simulink model "HilClimbers_Integrated_V8_2018b"  (R2018b)
settings: Solver=VariableStepAuto  StartTime=0.0  StopTime=20  RelTol=1e-3
undefined symbols (not defined in the file): air_conditioner_on_value, car_efficiency, op_type, sigbuilder_block, temperature_conversion, zero_check
libraries: BCM x10, simulink x2
settings Model: Creator=achu  LastModifiedBy=achu
settings DataIOCC: ReturnWorkspaceOutputs=on
settings DebuggingCC: AlgebraicLoopMsg=none  ParameterPrecisionLossMsg=none  SFMachineParentedDataDiag=error

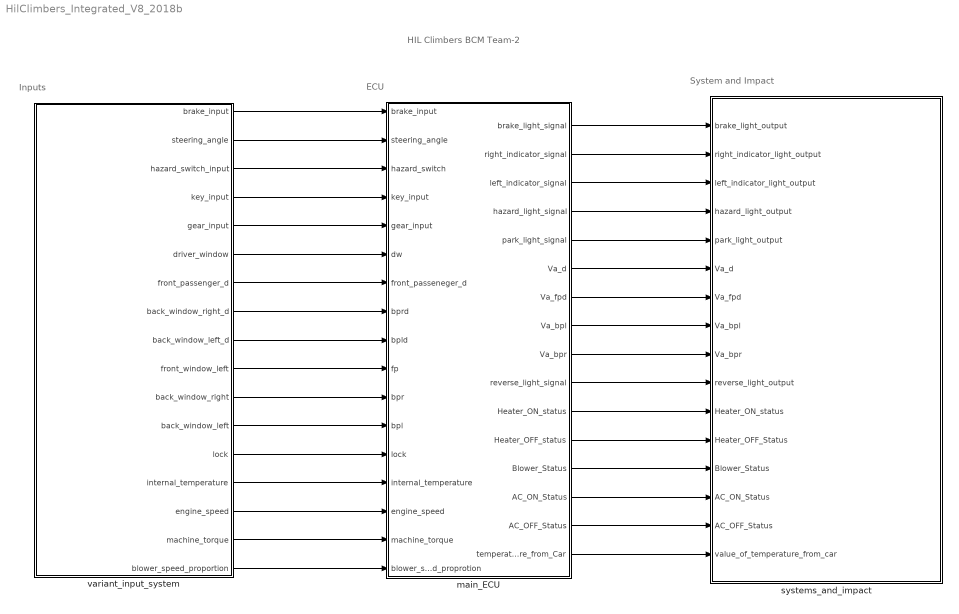
== system HilClimbers_Integrated_V8_2018b ==
  note: HIL Climbers BCM Team-2
  note: Inputs
  note: ECU
  note: System and Impact
  main_ECU : Subsystem
  systems_and_impact : Subsystem
  variant_input_system : Subsystem  Variant=on
  wires:
  main_ECU/3(left_indicator_signal) -> systems_and_impact/3(left_indicator_light_output)
  variant_input_system/13(lock) -> main_ECU/13(lock)
  variant_input_system/5(gear_input) -> main_ECU/5(gear_input)
  main_ECU/11(Heater_ON_status) -> systems_and_impact/11(Heater_ON_status)
  variant_input_system/9(back_window_left_d) -> main_ECU/9(bpld)
  variant_input_system/2(steering_angle) -> main_ECU/2(steering_angle)
  main_ECU/2(right_indicator_signal) -> systems_and_impact/2(right_indicator_light_output)
  variant_input_system/17(blower_speed_proportion) -> main_ECU/17(blower_speed_proprotion)
  main_ECU/16(temperature_from_Car) -> systems_and_impact/16(value_of_temperature_from_car)
  variant_input_system/12(back_window_left) -> main_ECU/12(bpl)
  main_ECU/15(AC_OFF_Status) -> systems_and_impact/15(AC_OFF_Status)
  variant_input_system/6(driver_window) -> main_ECU/6(dw)
  variant_input_system/7(front_passenger_d) -> main_ECU/7(front_passeneger_d)
  variant_input_system/16(machine_torque) -> main_ECU/16(machine_torque)
  main_ECU/4(hazard_light_signal) -> systems_and_impact/4(hazard_light_output)
  main_ECU/8(Va_bpl) -> systems_and_impact/8(Va_bpl)
  variant_input_system/15(engine_speed) -> main_ECU/15(engine_speed)
  main_ECU/10(reverse_light_signal) -> systems_and_impact/10(reverse_light_output)
  main_ECU/13(Blower_Status) -> systems_and_impact/13(Blower_Status)
  variant_input_system/3(hazard_switch_input) -> main_ECU/3(hazard_switch)
  main_ECU/14(AC_ON_Status) -> systems_and_impact/14(AC_ON_Status)
  variant_input_system/8(back_window_right_d) -> main_ECU/8(bprd)
  variant_input_system/14(internal_temperature) -> main_ECU/14(internal_temperature)
  variant_input_system/4(key_input) -> main_ECU/4(key_input)
  variant_input_system/1(brake_input) -> main_ECU/1(brake_input)
  main_ECU/6(Va_d) -> systems_and_impact/6(Va_d)
  variant_input_system/11(back_window_right) -> main_ECU/11(bpr)
  variant_input_system/10(front_window_left) -> main_ECU/10(fp)
  main_ECU/7(Va_fpd) -> systems_and_impact/7(Va_fpd)
  main_ECU/12(Heater_OFF_status) -> systems_and_impact/12(Heater_OFF_Status)
  main_ECU/1(brake_light_signal) -> systems_and_impact/1(brake_light_output)
  main_ECU/9(Va_bpr) -> systems_and_impact/9(Va_bpr)
  main_ECU/5(park_light_signal) -> systems_and_impact/5(park_light_output)

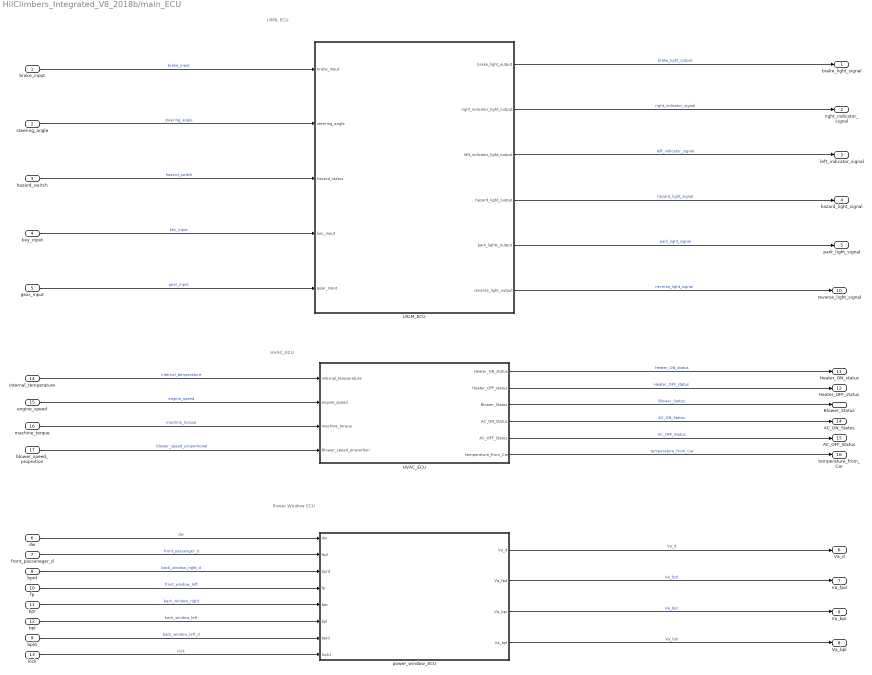
== system HilClimbers_Integrated_V8_2018b/main_ECU ==
  note: Power Window ECU
  note: HVAC_ECU
  note: LRML ECU
  brake_input : Inport
  steering_angle : Inport  Port=2
  hazard_switch : Inport  Port=3
  key_input : Inport  Port=4
  gear_input : Inport  Port=5
  dw : Inport  Port=6
  front_passeneger_d : Inport  Port=7
  bprd : Inport  Port=8
  bpld : Inport  Port=9
  fp : Inport  Port=10
  bpr : Inport  Port=11
  bpl : Inport  Port=12
  lock : Inport  Port=13
  internal_temperature : Inport  Port=14
  engine_speed : Inport  Port=15
  machine_torque : Inport  Port=16
  blower_speed_proprotion : Inport  Port=17
  HVAC_ECU : Subsystem
  LRLM_ECU : Subsystem
  power_window_ECU : Subsystem
  brake_light_signal : Outport
  right_indicator_signal : Outport  Port=2
  left_indicator_signal : Outport  Port=3
  hazard_light_signal : Outport  Port=4
  park_light_signal : Outport  Port=5
  Va_d : Outport  Port=6
  Va_fpd : Outport  Port=7
  Va_bpl : Outport  Port=8
  Va_bpr : Outport  Port=9
  reverse_light_signal : Outport  Port=10
  Heater_ON_status : Outport  Port=11
  Heater_OFF_status : Outport  Port=12
  Blower_Status : Outport  Port=13
  AC_ON_Status : Outport  Port=14
  AC_OFF_Status : Outport  Port=15
  temperature_from_Car : Outport  Port=16
  wires:
  HVAC_ECU/1(Heater_ON_status) -> Heater_ON_status/1  "Heater_ON_status"
  hazard_switch/1 -> LRLM_ECU/3(hazard_status)  "hazard_switch"
  LRLM_ECU/1(brake_light_output) -> brake_light_signal/1  "brake_light_output"
  HVAC_ECU/5(AC_OFF_Status) -> AC_OFF_Status/1  "AC_OFF_Status"
  steering_angle/1 -> LRLM_ECU/2(steering_angle)  "steering_angle"
  LRLM_ECU/2(right_indicator_light_output) -> right_indicator_signal/1  "right_indicator_signal"
  LRLM_ECU/5(park_lights_output) -> park_light_signal/1  "park_light_signal"
  brake_input/1 -> LRLM_ECU/1(brake_input)  "brake_input"
  engine_speed/1 -> HVAC_ECU/2(engine_speed)  "engine_speed"
  LRLM_ECU/3(left_indicator_light_output) -> left_indicator_signal/1  "left_indicator_signal"
  LRLM_ECU/4(hazard_light_output) -> hazard_light_signal/1  "hazard_light_signal"
  internal_temperature/1 -> HVAC_ECU/1(internal_temperature)  "internal_temperature"
  LRLM_ECU/6(reverse_light_output) -> reverse_light_signal/1  "reverse_light_signal"
  gear_input/1 -> LRLM_ECU/5(gear_input)  "gear_input"
  HVAC_ECU/2(Heater_OFF_status) -> Heater_OFF_status/1  "Heater_OFF_status"
  key_input/1 -> LRLM_ECU/4(key_input)  "key_input"
  blower_speed_proprotion/1 -> HVAC_ECU/4(Blower_speed_proportion)  "blower_speed_proportional"
  HVAC_ECU/6(temperature_from_Car) -> temperature_from_Car/1  "temperature_from_Car"
  HVAC_ECU/4(AC_ON_Status) -> AC_ON_Status/1  "AC_ON_Status"
  machine_torque/1 -> HVAC_ECU/3(machine_torque)  "machine_torque"
  HVAC_ECU/3(Blower_Status) -> Blower_Status/1  "Blower_Status"
  power_window_ECU/1(Va_d) -> Va_d/1  "Va_d"
  bpl/1 -> power_window_ECU/6(bpl)  "back_window_left"
  power_window_ECU/3(Va_bpr) -> Va_bpr/1  "Va_bpr"
  bpld/1 -> power_window_ECU/7(bpld)  "back_window_left_d"
  bprd/1 -> power_window_ECU/3(bprd)  "back_window_right_d"
  fp/1 -> power_window_ECU/4(fp)  "front_window_left"
  power_window_ECU/2(Va_fpd) -> Va_fpd/1  "Va_fpd"
  bpr/1 -> power_window_ECU/5(bpr)  "back_window_right"
  dw/1 -> power_window_ECU/1(dw)  "dw"
  power_window_ECU/4(Va_bpl) -> Va_bpl/1  "Va_bpl"
  lock/1 -> power_window_ECU/8(lock1)  "lock"
  front_passeneger_d/1 -> power_window_ECU/2(fpd)  "front_passenger_d"

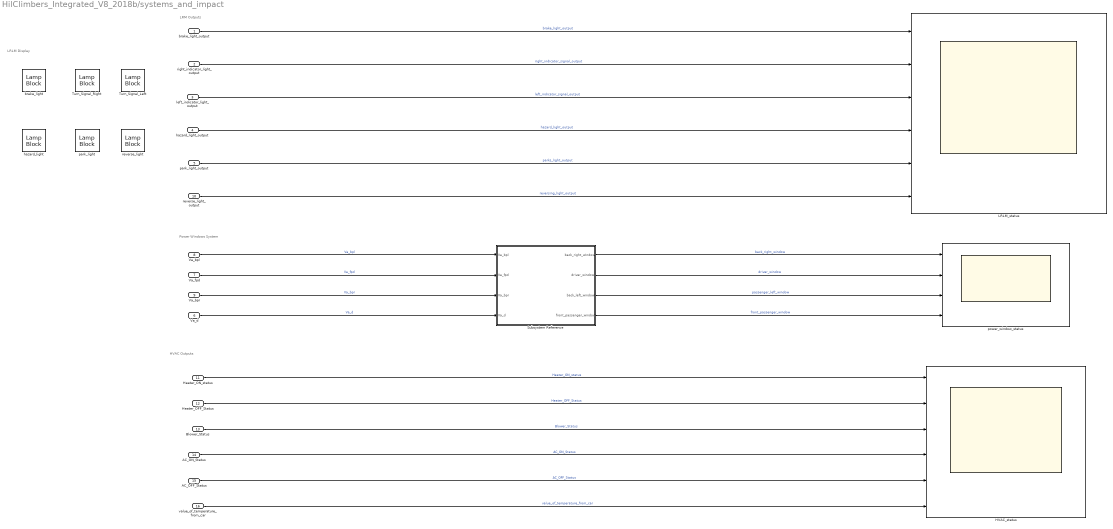
== system HilClimbers_Integrated_V8_2018b/systems_and_impact ==
  note: HVAC Outputs
  note: Power Windows System
  note: LRM Outputs
  note: LRLM Display
  brake_light_output : Inport
  right_indicator_light_output : Inport  Port=2
  left_indicator_light_output : Inport  Port=3
  hazard_light_output : Inport  Port=4
  park_light_output : Inport  Port=5
  Va_d : Inport  Port=6
  Va_fpd : Inport  Port=7
  Va_bpl : Inport  Port=8
  Va_bpr : Inport  Port=9
  reverse_light_output : Inport  Port=10
  Heater_ON_status : Inport  Port=11
  Heater_OFF_Status : Inport  Port=12
  Blower_Status : Inport  Port=13
  AC_ON_Status : Inport  Port=14
  AC_OFF_Status : Inport  Port=15
  value_of_temperature_from_car : Inport  Port=16
  HVAC_status : Scope  NumInputPorts=6
  LRLM_status : Scope  NumInputPorts=6
  Subsystem Reference : Subsystem
  Turn_Signal_Left : LampBlock  LabelPosition=Hide  Icon=TurnSignalLeft  WebBlockId=61
  Turn_Signal_Right : LampBlock  LabelPosition=Hide  Icon=TurnSignalRight  WebBlockId=62
  brake_light : LampBlock  LabelPosition=Hide  Icon=LightingSwitch  WebBlockId=63
  hazard_light : LampBlock  LabelPosition=Hide  Icon=Hazards  WebBlockId=64
  park_light : LampBlock  LabelPosition=Hide  Icon=ParkingAssistance  WebBlockId=65
  power_window_status : Scope  NumInputPorts=4
  reverse_light : LampBlock  LabelPosition=Hide  Icon=RearFogLight  WebBlockId=67
  wires:
  hazard_light_output/1 -> LRLM_status/4  "hazard_light_output"
  reverse_light_output/1 -> LRLM_status/6  "reversing_light_output"
  park_light_output/1 -> LRLM_status/5  "parks_light_output"
  left_indicator_light_output/1 -> LRLM_status/3  "left_indicator_signal_output"
  right_indicator_light_output/1 -> LRLM_status/2  "right_indicator_signal_output"
  brake_light_output/1 -> LRLM_status/1  "brake_light_output"
  Subsystem Reference/4(front_passenger_window) -> power_window_status/4  "front_passenger_window"
  Subsystem Reference/3(back_left_window) -> power_window_status/3  "passenger_left_window"
  Subsystem Reference/1(back_right_window) -> power_window_status/1  "back_right_window"
  Subsystem Reference/2(driver_window) -> power_window_status/2  "driver_window"
  Blower_Status/1 -> HVAC_status/3  "Blower_Status"
  AC_OFF_Status/1 -> HVAC_status/5  "AC_OFF_Status"
  AC_ON_Status/1 -> HVAC_status/4  "AC_ON_Status"
  Heater_OFF_Status/1 -> HVAC_status/2  "Heater_OFF_Status"
  Heater_ON_status/1 -> HVAC_status/1  "Heater_ON_status"
  value_of_temperature_from_car/1 -> HVAC_status/6  "value_of_temperature_from_car"
  Va_bpl/1 -> Subsystem Reference/1(Va_bpl)  "Va_bpl"
  Va_fpd/1 -> Subsystem Reference/2(Va_fpd)  "Va_fpd"
  Va_d/1 -> Subsystem Reference/4(Va_d)  "Va_d"
  Va_bpr/1 -> Subsystem Reference/3(Va_bpr)  "Va_bpr"

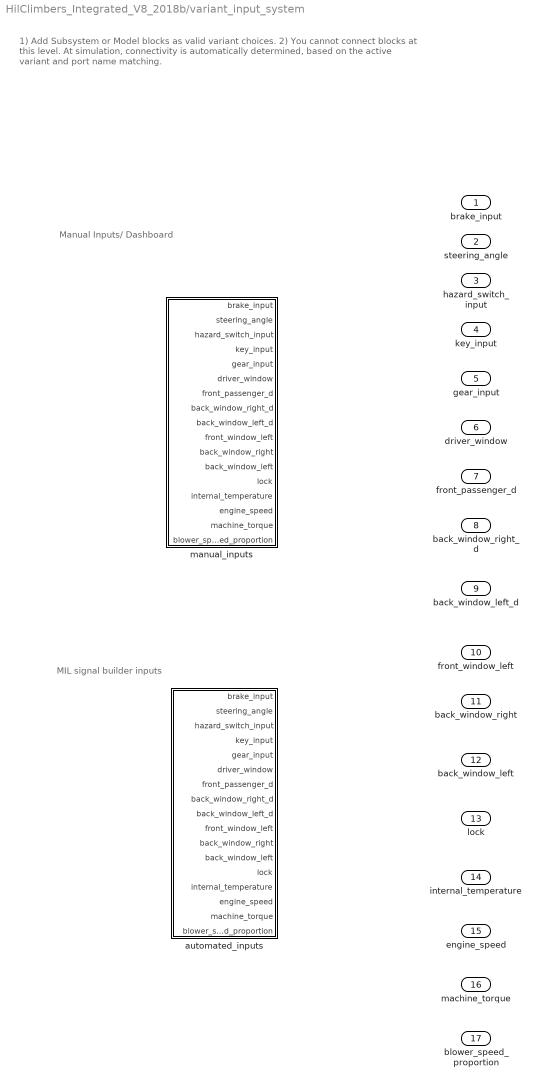
== system HilClimbers_Integrated_V8_2018b/variant_input_system ==
  note: MIL signal builder inputs
  note: Manual Inputs/ Dashboard
  note: 1) Add Subsystem or Model blocks as valid variant choices.
      | 2) You cannot connect blocks at this level. At simulation, connectivity is automatically
      | determined, based on the active variant and port name matching.
  automated_inputs : Subsystem  VariantControl=automated_input
  manual_inputs : Subsystem  VariantControl=manual_input
  brake_input : Outport
  steering_angle : Outport  Port=2
  hazard_switch_input : Outport  Port=3
  key_input : Outport  Port=4
  gear_input : Outport  Port=5
  driver_window : Outport  Port=6
  front_passenger_d : Outport  Port=7
  back_window_right_d : Outport  Port=8
  back_window_left_d : Outport  Port=9
  front_window_left : Outport  Port=10
  back_window_right : Outport  Port=11
  back_window_left : Outport  Port=12
  lock : Outport  Port=13
  internal_temperature : Outport  Port=14
  engine_speed : Outport  Port=15
  machine_torque : Outport  Port=16
  blower_speed_proportion : Outport  Port=17

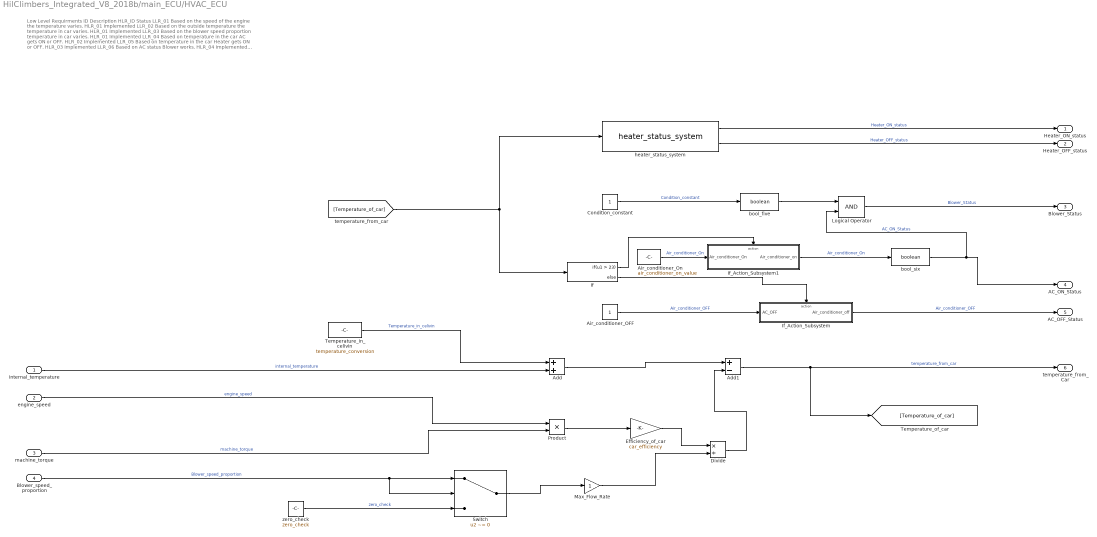
== system HilClimbers_Integrated_V8_2018b/main_ECU/HVAC_ECU ==
  note: Low Level Requirments
      | ID
      | Description
      | HLR_ID
      | Status
      |
      | LLR_01
      | Based on the speed of the engine the temperature varies.
      | HLR_01
      | Implemented
      |
      | LLR_02
      | Based on the outside temperature the temperature in car varies.
      | HLR_01
      | Implemented
      |
      | LLR_03
      | Based on the blower speed proportion temperature in car varies.
      | HLR_01
      | Implemented
      |
      | LLR_04
      | Based on temperature in the car AC gets ON or OFF.
      | HLR_02
      | Implemented
      |
      | LLR_05
      | Based on temperature in the car Heater gets ON or OFF.
      | HLR_03
      | Implemented
      |
      | LLR_06
      | Based on AC status Blower works.
      | HLR_04
      | Implemented
      |
      | LOGIC:
      | STEP 1. Taking values of engine temperature and comp Torque and multipled and given to efficiency(gain).
      | STEP 2. Blower speed proportion and given toMaximum flow rate(gain).
      | STEP 3. Both values were given to divide block.
      | STEP 4. Internal Temperature is in degrees and after it converted into kelvin.
      | STEP 5. Subtract of both values, then the temperature will display on the Display block.
      | 1.Based on temperature the AC is getting on.
      | a.If the value(temperature) is greater than 23 then AC should be on.
      | b.Else the AC should be off.
      | 2. Based on AC status Blower Works.
      | 3. Based on temperature the Blower is getting on.
      | a.If the value(temperature) is less than 18 then Heater should be on.
      | b.Else the Heater should be off.
  internal_temperature : Inport
  engine_speed : Inport  Port=2
  machine_torque : Inport  Port=3
  Blower_speed_proportion : Inport  Port=4
  Add : Sum
  Add1 : Sum  Inputs=+-
  Air_conditioner_OFF : Constant
  Air_conditioner_On : Constant  Value=air_conditioner_on_value
  Condition_constant : Constant
  Divide : Product  Inputs=*/
  Efficiency_of_car : Gain  Gain=car_efficiency
  If : If  IfExpression=u1 > 23
  If_Action_Subsystem : Subsystem  TreatAsAtomicUnit=on
  If_Action_Subsystem1 : Subsystem  TreatAsAtomicUnit=on
  Logical Operator : Logic  AllPortsSameDT=off  OutDataTypeStr=boolean
  Max_Flow_Rate : Gain
  Product : Product
  Switch : Switch  Criteria=u2 ~= 0
  Temperature_in_celivin : Constant  Value=temperature_conversion
  bool_five : DataTypeConversion  OutDataTypeStr=boolean
  bool_six : DataTypeConversion  OutDataTypeStr=boolean
  heater_status_system : BCM/heater_status_system  SystemSampleTime=-1  Latency=0  AutoFrameSizeCalculation=off
      settings: SourceProductName=BCM Library
  zero_check : Constant  Value=zero_check
  Heater_ON_status : Outport
  Heater_OFF_status : Outport  Port=2
  Blower_Status : Outport  Port=3
  AC_ON_Status : Outport  Port=4
  AC_OFF_Status : Outport  Port=5
  temperature_from_Car : Outport  Port=6
  wires:
  Add1/1 -> temperature_from_Car/1, [Temperature_of_car]  "temperature_from_car"
  If_Action_Subsystem/1(Air_conditioner_off) -> AC_OFF_Status/1  "Air_conditioner_OFF"
  Divide/1 -> Add1/2
  [Temperature_of_car] -> heater_status_system/1, If/1
  Condition_constant/1 -> bool_five/1  "Condition_constant"
  Efficiency_of_car/1 -> Divide/1
  If/1 -> If_Action_Subsystem1/Action
  Air_conditioner_OFF/1 -> If_Action_Subsystem/1(AC_OFF)  "Air_conditioner_OFF"
  Max_Flow_Rate/1 -> Divide/2
  Add/1 -> Add1/1
  Temperature_in_celivin/1 -> Add/1  "Temperature_in_celivin"
  engine_speed/1 -> Product/1  "engine_speed"
  machine_torque/1 -> Product/2  "machine_torque"
  internal_temperature/1 -> Add/2  "internal_temperature"
  If/2 -> If_Action_Subsystem/Action
  Product/1 -> Efficiency_of_car/1
  Logical Operator/1 -> Blower_Status/1  "Blower_Status"
  Air_conditioner_On/1 -> If_Action_Subsystem1/1(Air_conditioner_On)  "Air_conditioner_On"
  heater_status_system/1 -> Heater_ON_status/1  "Heater_ON_status"
  heater_status_system/2 -> Heater_OFF_status/1  "Heater_OFF_status"
  Switch/1 -> Max_Flow_Rate/1
  Blower_speed_proportion/1 -> Switch/1, Switch/2  "Blower_speed_proportion"
  bool_five/1 -> Logical Operator/1
  If_Action_Subsystem1/1(Air_conditioner_on) -> bool_six/1  "Air_conditioner_On"
  bool_six/1 -> Logical Operator/2, AC_ON_Status/1  "AC_ON_Status"
  zero_check/1 -> Switch/3  "zero_check"

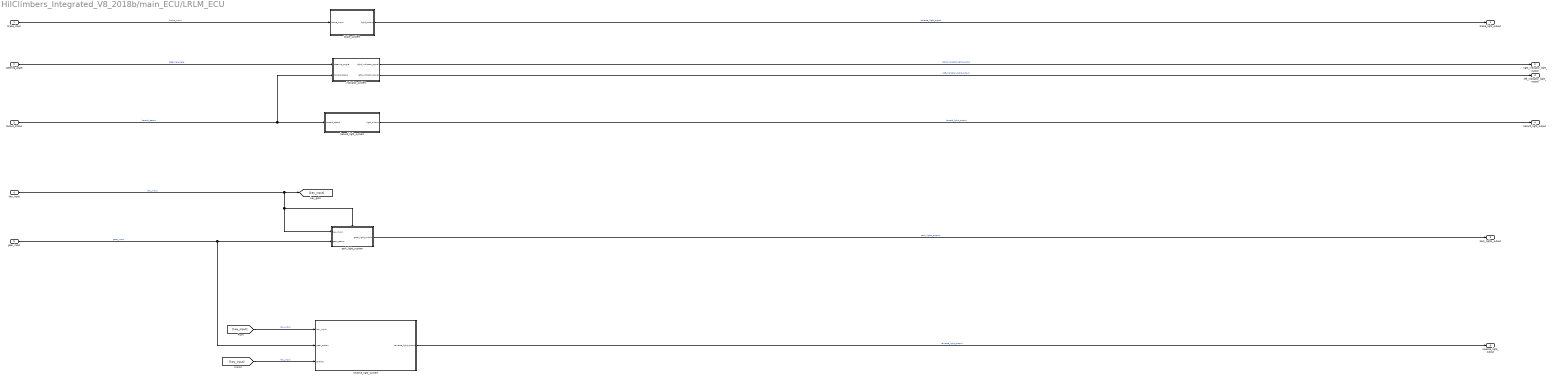
== system HilClimbers_Integrated_V8_2018b/main_ECU/LRLM_ECU ==
  brake_input : Inport
  steering_angle : Inport  Port=2
  hazard_status : Inport  Port=3
  key_input : Inport  Port=4
  gear_input : Inport  Port=5
  brake_system : Subsystem  TreatAsAtomicUnit=on
      mask Display: disp("Brake System");
  hazard_light_system : Subsystem
  indicator_system : Subsystem  TreatAsAtomicUnit=on
  park_light_system : Subsystem
  reverse_light_system : Subsystem  Variant=on
  brake_light_output : Outport
  right_indicator_light_output : Outport  Port=2
  left_indicator_light_output : Outport  Port=3
  hazard_light_output : Outport  Port=4
  park_lights_output : Outport  Port=5
  reverse_light_output : Outport  Port=6
  wires:
  hazard_light_system/1(light_output) -> hazard_light_output/1  "hazard_light_output"
  brake_input/1 -> brake_system/1(brake_input)  "brake_input"
  park_light_system/1(gear_light_output) -> park_lights_output/1  "park_lights_output"
  hazard_status/1 -> indicator_system/2(hazard_status), hazard_light_system/1(hazard_status)  "hazard_status"
  indicator_system/2(left_indicator_signal) -> left_indicator_light_output/1  "left_indicator_light_output"
  indicator_system/1(right_indicator_signal) -> right_indicator_light_output/1  "right_indicator_light_output"
  steering_angle/1 -> indicator_system/1(steering_angle)  "steering_angle"
  brake_system/1(light_output) -> brake_light_output/1  "reverse_light_signal"
  gear_input/1 -> reverse_light_system/2(gear_option), park_light_system/2(gear_status)  "gear_input"
  key_input/1 -> park_light_system/Enable, park_light_system/1(key_input), [key_input]  "key_input"
  [key_input] -> reverse_light_system/1(key_input)  "key_input"
  [key_input] -> reverse_light_system/3(Enable)  "key_input"
  reverse_light_system/1(reverse_light_output) -> reverse_light_output/1  "reverse_light_output"

== system HilClimbers_Integrated_V8_2018b/main_ECU/power_window_ECU ==
  dw : Inport
  fpd : Inport  Port=2
  bprd : Inport  Port=3
  fp : Inport  Port=4
  bpr : Inport  Port=5
  bpl : Inport  Port=6
  bpld : Inport  Port=7
  lock1 : Inport  Port=8
  Checking_priority : Subsystem  TreatAsAtomicUnit=on
  MATLAB Function4 : MATLAB Function  TreatAsAtomicUnit=on
  Va_d : Outport
  Va_fpd : Outport  Port=2
  Va_bpr : Outport  Port=3
  Va_bpl : Outport  Port=4
  wires:
  MATLAB Function4/2(Va_fpd) -> Va_fpd/1  "Va_fpd"
  MATLAB Function4/3(Va_bpr) -> Va_bpr/1  "Va_bpr"
  lock1/1 -> Checking_priority/5(lock)  "lock"
  fpd/1 -> Checking_priority/1(fpd)  "fpd"
  bpld/1 -> Checking_priority/4(bpld)  "bpld"
  MATLAB Function4/1(Va_d) -> Va_d/1  "Va_d"
  Checking_priority/1(front_passenger) -> MATLAB Function4/2(front_passenger)  "front_passenger"
  dw/1 -> MATLAB Function4/1(dw)  "dw"
  bpl/1 -> Checking_priority/3(bpl)  "bpl"
  Checking_priority/2(back_passenger_right) -> MATLAB Function4/3(back_passenger_right)  "back_passenger_right"
  fp/1 -> Checking_priority/7(fp)  "fp"
  bpr/1 -> Checking_priority/6(bpr)  "bpr"
  bprd/1 -> Checking_priority/2(bprd)  "bprd"
  Checking_priority/3(back_passenger_left) -> MATLAB Function4/4(back_passenger_left)  "back_passenger_left"
  MATLAB Function4/4(Va_bpl) -> Va_bpl/1  "Va_bpl"

== system HilClimbers_Integrated_V8_2018b/systems_and_impact/Subsystem Reference ==
  Va_bpl : Inport
  Va_fpd : Inport  Port=2
  Va_bpr : Inport  Port=3
  Va_d : Inport  Port=4
  MATLAB Function : MATLAB Function  TreatAsAtomicUnit=on
  power_window_dc_motor{,1..3} (4 alike) : BCM/power_window_dc_motor  SystemSampleTime=-1  Latency=0  AutoFrameSizeCalculation=off
      settings: SourceProductName=BCM Library
  back_right_window : Outport
  driver_window : Outport  Port=2
  back_left_window : Outport  Port=3
  front_passenger_window : Outport  Port=4
  wires:
  Va_fpd/1 -> power_window_dc_motor3/2, power_window_dc_motor3/1  "Va_fpd"
  Va_d/1 -> power_window_dc_motor1/2, power_window_dc_motor1/1  "Va_d"
  power_window_dc_motor3/1 -> MATLAB Function/4(fp)
  power_window_dc_motor1/1 -> MATLAB Function/2(d)  "d"
  MATLAB Function/1(pr_o) -> back_right_window/1  "back_right_window"
  power_window_dc_motor/1 -> MATLAB Function/1(pr)
  Va_bpr/1 -> power_window_dc_motor/2, power_window_dc_motor/1  "Va_bpr"
  MATLAB Function/2(d_o) -> driver_window/1  "driver_window"
  MATLAB Function/3(pl_o) -> back_left_window/1  "back_left_window"
  MATLAB Function/4(fp_o) -> front_passenger_window/1  "front_passenger_window"
  Va_bpl/1 -> power_window_dc_motor2/2, power_window_dc_motor2/1  "Va_bpl"
  power_window_dc_motor2/1 -> MATLAB Function/3(pl)  "d"

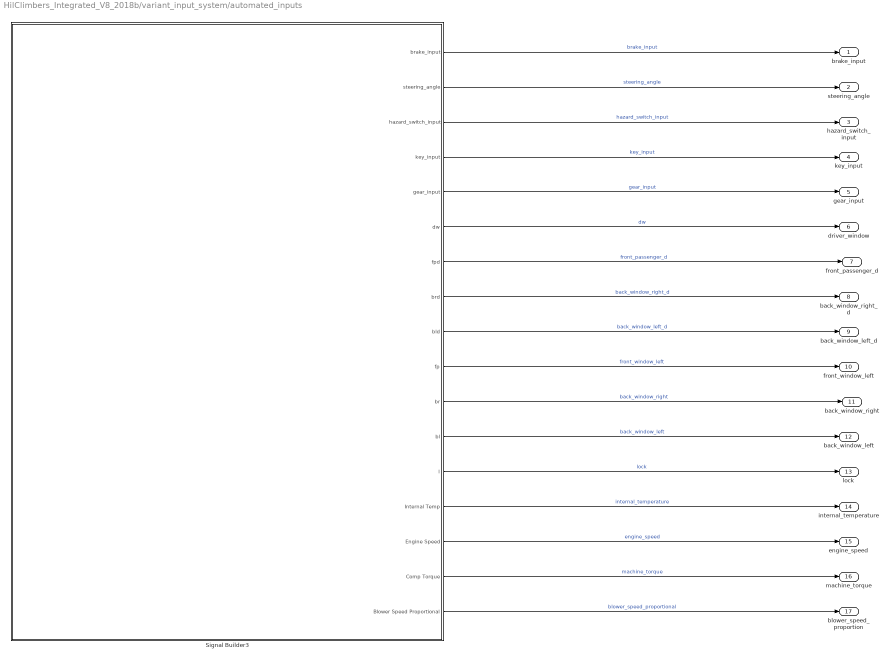
== system HilClimbers_Integrated_V8_2018b/variant_input_system/automated_inputs ==
  Signal Builder3 : Subsystem  Tag=STV Subsys  LoadFcn=sigbuilder_block('load');  StartFcn=sigbuilder_block('start');  StopFcn=sigbuilder_block('stop');  ClipboardFcn=sigbuilder_block('clipboard');  mask(Sigbuilder block){tuvar=[0:10]}
      mask help: Simulink:masks:SigbuilderBlock_MD
      mask init:
      | if ~strcmp(get_param(bdroot(gcbh),'SimulationStatus'),'stopped') tuvar = sigbuilder_block('maskInit'); end
      settings: CopyFcn=sigbuilder_block('copy');  DeleteFcn=sigbuilder_block('delete');  ModelCloseFcn=sigbuilder_block('modelClose');  PreSaveFcn=sigbuilder_block('preSave');  PauseFcn=sigbuilder_block('pause');  ContinueFcn=sigbuilder_block('continue');  NameChangeFcn=sigbuilder_block('namechange');  OpenFcn=sigbuilder_block('open',[437.6 199.2 550.4 400 ]);  CloseFcn=sigbuilder_block('close');
      mask Display: plot(0, 0, 100, 100,[2, 2, 32, 32, 2], [68, 8, 8, 68, 68],[32, 2], [38, 38], [32, 19, 2],[53, 60, 44], [32, 17, 17, 2],[16, 16, 31, 31]);txt = getActiveGroup(gcbh);text(2, 100, txt,'verticalAlignment', 'top');
  brake_input : Outport
  steering_angle : Outport  Port=2
  hazard_switch_input : Outport  Port=3
  key_input : Outport  Port=4
  gear_input : Outport  Port=5
  driver_window : Outport  Port=6
  front_passenger_d : Outport  Port=7
  back_window_right_d : Outport  Port=8
  back_window_left_d : Outport  Port=9
  front_window_left : Outport  Port=10
  back_window_right : Outport  Port=11
  back_window_left : Outport  Port=12
  lock : Outport  Port=13
  internal_temperature : Outport  Port=14
  engine_speed : Outport  Port=15
  machine_torque : Outport  Port=16
  blower_speed_proportion : Outport  Port=17
  wires:
  Signal Builder3/11(br) -> back_window_right/1  "back_window_right"
  Signal Builder3/2(steering_angle) -> steering_angle/1  "steering_angle"
  Signal Builder3/13(l) -> lock/1  "lock"
  Signal Builder3/16(Comp Torque) -> machine_torque/1  "machine_torque"
  Signal Builder3/10(fp) -> front_window_left/1  "front_window_left"
  Signal Builder3/5(gear_input) -> gear_input/1  "gear_input"
  Signal Builder3/12(bl) -> back_window_left/1  "back_window_left"
  Signal Builder3/17(Blower Speed Proportional) -> blower_speed_proportion/1  "blower_speed_proportional"
  Signal Builder3/8(brd) -> back_window_right_d/1  "back_window_right_d"
  Signal Builder3/14(Internal Temp) -> internal_temperature/1  "internal_temperature"
  Signal Builder3/3(hazard_switch_input) -> hazard_switch_input/1  "hazard_switch_input"
  Signal Builder3/6(dw) -> driver_window/1  "dw"
  Signal Builder3/1(brake_input) -> brake_input/1  "brake_input"
  Signal Builder3/7(fpd) -> front_passenger_d/1  "front_passenger_d"
  Signal Builder3/9(bld) -> back_window_left_d/1  "back_window_left_d"
  Signal Builder3/15(Engine Speed) -> engine_speed/1  "engine_speed"
  Signal Builder3/4(key_input) -> key_input/1  "key_input"

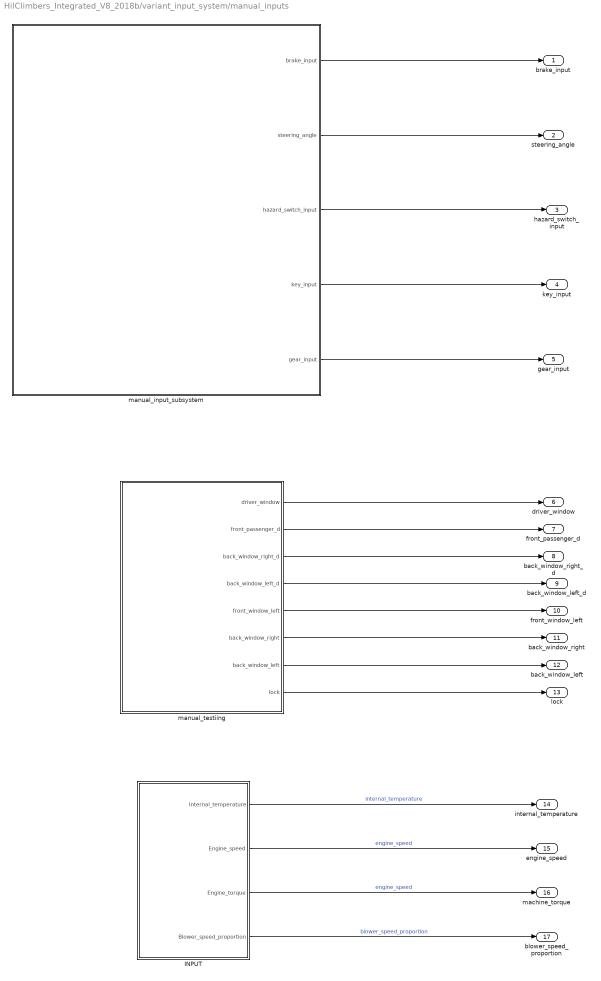
== system HilClimbers_Integrated_V8_2018b/variant_input_system/manual_inputs ==
  INPUT : Subsystem
  manual_input_subsystem : Subsystem  VariantControl=manual_test
  manual_testiing : Subsystem  VariantControl=Choice
  brake_input : Outport
  steering_angle : Outport  Port=2
  hazard_switch_input : Outport  Port=3
  key_input : Outport  Port=4
  gear_input : Outport  Port=5
  driver_window : Outport  Port=6
  front_passenger_d : Outport  Port=7
  back_window_right_d : Outport  Port=8
  back_window_left_d : Outport  Port=9
  front_window_left : Outport  Port=10
  back_window_right : Outport  Port=11
  back_window_left : Outport  Port=12
  lock : Outport  Port=13
  internal_temperature : Outport  Port=14
  engine_speed : Outport  Port=15
  machine_torque : Outport  Port=16
  blower_speed_proportion : Outport  Port=17
  wires:
  manual_input_subsystem/3(hazard_switch_input) -> hazard_switch_input/1
  manual_input_subsystem/2(steering_angle) -> steering_angle/1
  manual_input_subsystem/4(key_input) -> key_input/1
  manual_testiing/1(driver_window) -> driver_window/1
  manual_input_subsystem/1(brake_input) -> brake_input/1
  manual_testiing/6(back_window_right) -> back_window_right/1
  manual_testiing/5(front_window_left) -> front_window_left/1
  manual_input_subsystem/5(gear_input) -> gear_input/1
  manual_testiing/3(back_window_right_d) -> back_window_right_d/1
  INPUT/1(Internal_temperature) -> internal_temperature/1  "internal_temperature"
  manual_testiing/8(lock) -> lock/1
  INPUT/3(Engine_torque) -> machine_torque/1  "engine_speed"
  manual_testiing/4(back_window_left_d) -> back_window_left_d/1
  INPUT/2(Engine_speed) -> engine_speed/1  "engine_speed"
  manual_testiing/2(front_passenger_d) -> front_passenger_d/1
  INPUT/4(Blower_speed_proportion) -> blower_speed_proportion/1  "blower_speed_proportion"
  manual_testiing/7(back_window_left) -> back_window_left/1

== system HilClimbers_Integrated_V8_2018b/main_ECU/HVAC_ECU/If_Action_Subsystem ==
  AC_OFF : Inport
  Action_Port : ActionPort
  Air_conditioner_off : Outport
  wires:
  AC_OFF/1 -> Air_conditioner_off/1  "AC_OFF"

== system HilClimbers_Integrated_V8_2018b/main_ECU/HVAC_ECU/If_Action_Subsystem1 ==
  Air_conditioner_On : Inport
  Action_Port : ActionPort
  Air_conditioner_on : Outport
  wires:
  Air_conditioner_On/1 -> Air_conditioner_on/1  "Air_conditioner_On"

== system HilClimbers_Integrated_V8_2018b/main_ECU/LRLM_ECU/brake_system ==
  brake_input : Inport
  brake/hazard_light_output_decider : BCM/brake//hazard_light_output_decider
      settings: SourceProductName=BCM Library
  light_output : Outport
  wires:
  brake_input/1 -> brake/hazard_light_output_decider/1  "brake_input"
  brake/hazard_light_output_decider/1 -> light_output/1

== system HilClimbers_Integrated_V8_2018b/main_ECU/LRLM_ECU/hazard_light_system ==
  hazard_status : Inport
  brake/hazard_light_output_decider : BCM/brake//hazard_light_output_decider
      settings: SourceProductName=BCM Library
  light_output : Outport
  wires:
  brake/hazard_light_output_decider/1 -> light_output/1  "light_output"
  hazard_status/1 -> brake/hazard_light_output_decider/1  "hazard_switch_input"

== system HilClimbers_Integrated_V8_2018b/main_ECU/LRLM_ECU/indicator_system ==
  steering_angle : Inport
  hazard_status : Inport  Port=2
  left_indicator_system : Subsystem
  right_indicator_system : Subsystem
  right_indicator_signal : Outport
  left_indicator_signal : Outport  Port=2
  wires:
  left_indicator_system/1(left_indicator_signal) -> left_indicator_signal/1  "left_indicator_signal"
  right_indicator_system/1(right_indicator_signal) -> right_indicator_signal/1  "right_indicator_signal"
  hazard_status/1 -> right_indicator_system/2(hazard_status), left_indicator_system/2(hazard_status)  "hazard_status"
  steering_angle/1 -> right_indicator_system/1(steering_angle), [steering_angle]  "steering_angle"
  [steering_angle] -> left_indicator_system/1(steering_angle)  "steering_angle"

== system HilClimbers_Integrated_V8_2018b/main_ECU/LRLM_ECU/park_light_system ==
  key_input : Inport
  gear_status : Inport  Port=2
  Enable : EnablePort  StatesWhenEnabling=reset
  bool_fourty : DataTypeConversion  OutDataTypeStr=boolean
  bool_fourtyone : DataTypeConversion  OutDataTypeStr=boolean
  park_gear_lights_output_decider : BCM/reverse//park_gear_lights_output_decider  gear_option=Park
      settings: SourceProductName=BCM Library
  gear_light_output : Outport
  wires:
  bool_fourty/1 -> park_gear_lights_output_decider/1
  bool_fourtyone/1 -> park_gear_lights_output_decider/2
  key_input/1 -> bool_fourty/1  "key_input"
  gear_status/1 -> bool_fourtyone/1  "gear_status"
  park_gear_lights_output_decider/1 -> gear_light_output/1  "gear_light_output"

== system HilClimbers_Integrated_V8_2018b/main_ECU/LRLM_ECU/reverse_light_system ==
  note: 1) Add Subsystem or Model blocks as valid variant choices.
      | 2) You cannot connect blocks at this level. At simulation, connectivity is automatically
      | determined, based on the active variant and port name matching.
  key_input : Inport
  gear_option : Inport  Port=2
  Enable : Inport  Port=3
  reverse_light_mil : Subsystem  TreatAsAtomicUnit=on  VariantControl=reverse_light_sys_mil  mask{out_type=Reverse lights will blink}
      mask prompts: out_type "Enter the mode of reverse lights"
      mask init:
      | assignin('base','op_type',out_type);
      mask TypeOptions out_type: Reverse lights will blink | Reverse lights will not blink
  reverse_light_sil : Subsystem  VariantControl=reverse_light_sys_sil  mask{sfcnParam1=op_type}
      mask prompts: sfcnParam1 "op_type:"
      mask help: Simulink:masks:GenSFuncDesc_MD
      mask Help: eval('feval(''rtwprivate'',''rtwhelpview'',''rtw_sfcn_block'')');
  reverse_light_output : Outport

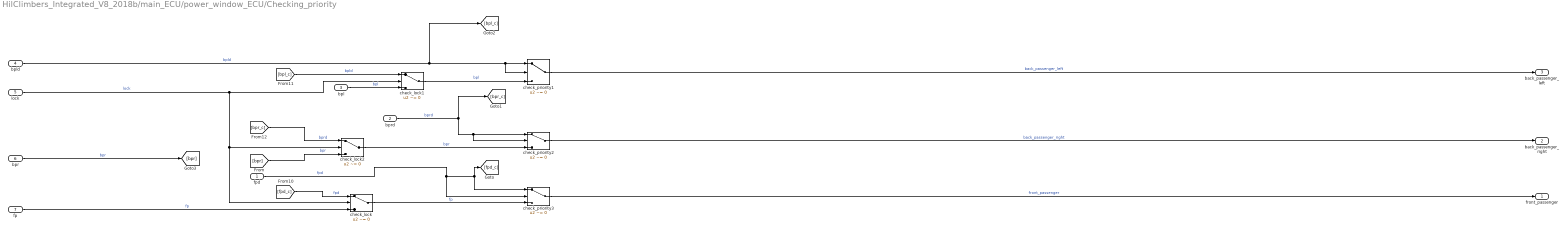
== system HilClimbers_Integrated_V8_2018b/main_ECU/power_window_ECU/Checking_priority ==
  fpd : Inport
  bprd : Inport  Port=2
  bpl : Inport  Port=3
  bpld : Inport  Port=4
  lock : Inport  Port=5
  bpr : Inport  Port=6
  fp : Inport  Port=7
  check_lock : Switch  Criteria=u2 ~= 0
  check_lock1 : Switch  Criteria=u2 ~= 0
  check_lock2 : Switch  Criteria=u2 ~= 0
  check_priority1 : Switch  Criteria=u2 ~= 0
  check_priority2 : Switch  Criteria=u2 ~= 0
  check_priority3 : Switch  Criteria=u2 ~= 0
  front_passenger : Outport
  back_passenger_right : Outport  Port=2
  back_passenger_left : Outport  Port=3
  wires:
  check_lock2/1 -> check_priority2/3  "bpr"
  bprd/1 -> check_priority2/2, check_priority2/1, [bpr_c]  "bprd"
  bpld/1 -> [bpl_c], check_priority1/1, check_priority1/2  "bpld"
  check_priority1/1 -> back_passenger_left/1  "back_passenger_left"
  check_priority2/1 -> back_passenger_right/1  "back_passenger_right"
  check_priority3/1 -> front_passenger/1  "front_passenger"
  lock/1 -> check_lock/2, check_lock2/2, check_lock1/2  "lock"
  bpl/1 -> check_lock1/3  "bpl"
  check_lock1/1 -> check_priority1/3  "bpl"
  [bpl_c] -> check_lock1/1  "bpld"
  [fpd_c] -> check_lock/1  "fpd"
  [bpr] -> check_lock2/3  "bpr"
  [bpr_c] -> check_lock2/1  "bprd"
  bpr/1 -> [bpr]  "bpr"
  fp/1 -> check_lock/3  "fp"
  fpd/1 -> check_priority3/2, [fpd_c], check_priority3/1  "fpd"
  check_lock/1 -> check_priority3/3  "fp"

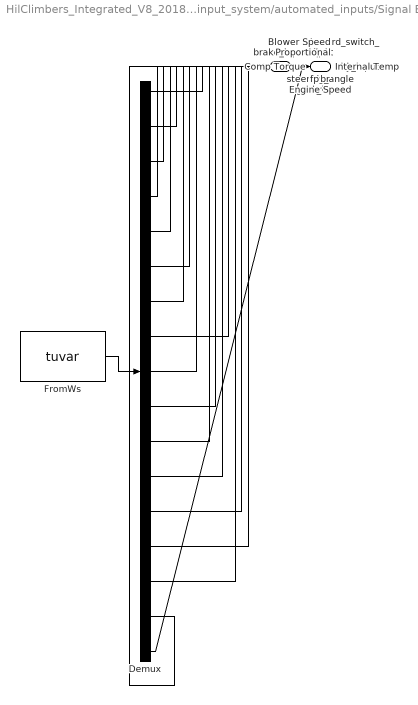
== system HilClimbers_Integrated_V8_2018b/variant_input_system/automated_inputs/Signal Builder3 ==
  Demux : Demux  Tag=STV Demux  Outputs=17
      settings: DisplayOption=none
  FromWs : FromWorkspace  Tag=STV FromWs  VariableName=tuvar
      SigBuilderData=|
      | common.afterFinalStr = 'Extrapolate'
      | common.sampleTime = 0
      | dataSet.timeRange = [0 20]
      | dataSet.name = 'Sheet1'
      | sbobj.Name = 'Signal Builder'
      | sbobj.Groups.Name = 'Sheet1'
      | sbobj.Groups.Signals(1).Name = 'brake_input'
      | sbobj.Groups.Signals(1).XData = [0 1 2 3 4 5 6 7 8 9 10 11 12 13 14 15 16 17 18 19 20]
      | sbobj.Groups.Signals(1).YData = [0 0 0 0 0 0 0 0 0 0 0 1 1 1 1 1 1 1 1 1 1]
      | sbobj.Groups.Signals(2).Name = 'steering_angle'
      | sbobj.Groups.Signals(2).XData = [0 1 2 3 4 5 6 7 8 9 10 11 12 13 14 15 16 17 18 19 20]
      | sbobj.Groups.Signals(2).YData = [-45 -45 -45 -45 -45 -45 -45 -45 0 0 0 0 0 0 0 0 45 45 45 45 45]
      | sbobj.Groups.Signals(3).Name = 'hazard_switch_input'
      | sbobj.Groups.Signals(3).XData = [0 1 2 3 4 5 6 7 8 9 10 11 12 13 14 15 16 17 18 19 20]
      | sbobj.Groups.Signals(3).YData = [0 0 0 0 0 0 0 0 0 0 0 0 0 0 0 0 1 1 1 1 1]
      | sbobj.Groups.Signals(4).Name = 'key_input'
      | sbobj.Groups.Signals(4).XData = [0 1 2 3 4 5 6 7 8 9 10 11 12 13 14 15 16 17 18 19 20]
      | sbobj.Groups.Signals(4).YData = [0 0 0 0 0 0 0 0 1 1 1 1 1 1 1 1 0 0 0 0 0]
      | sbobj.Groups.Signals(5).Name = 'gear_input'
      | sbobj.Groups.Signals(5).XData = [0 1 2 3 4 5 6 7 8 9 10 11 12 13 14 15 16 17 18 19 20]
      | sbobj.Groups.Signals(5).YData = [0 0 1 1 2 2 3 3 0 0 1 1 2 2 3 3 0 0 1 1 1]
      | sbobj.Groups.Signals(6).Name = 'dw'
      | sbobj.Groups.Signals(6).XData = [0 1 2 3 4 5 6 7 8 9 10 11 12 13 14 15 16 17 18 19 20]
      | sbobj.Groups.Signals(6).YData = [0 0 1 1 1 1 1 1 1 1 1 0 0 0 0 -1 -1 -1 -1 -1 -1]
      | sbobj.Groups.Signals(7).Name = 'fpd'
      | sbobj.Groups.Signals(7).XData = [0 1 2 3 4 5 6 7 8 9 10 11 12 13 14 15 16 17 18 19 20]
      | sbobj.Groups.Signals(7).YData = [0 0 1 -1 -1 1 1 1 1 1 1 1 1 1 1 1 0 0 0 0 0]
      | sbobj.Groups.Signals(8).Name = 'brd'
      | sbobj.Groups.Signals(8).XData = [0 1 2 3 4 5 6 7 8 9 10 11 12 13 14 15 16 17 18 19 20]
      | sbobj.Groups.Signals(8).YData = [0 0 1 1 1 1 1 1 -1 -1 -1 0 0 0 0 0 0 0 0 0 0]
      | sbobj.Groups.Signals(9).Name = 'bld'
      | sbobj.Groups.Signals(9).XData = [0 1 2 3 4 5 6 7 8 9 10 11 12 13 14 15 16 17 18 19 20]
      | sbobj.Groups.Signals(9).YData = [0 0 1 1 1 1 1 1 1 1 1 0 0 0 0 0 0 0 0 0 0]
      | sbobj.Groups.Signals(10).Name = 'fp'
      | sbobj.Groups.Signals(10).XData = [0 1 2 3 4 5 6 7 8 9 10 11 12 13 14 15 16 17 18 19 20]
      | sbobj.Groups.Signals(10).YData = [0 -1 -1 1 1 1 -1 -1 -1 -1 -1 -1 -1 -1 1 1 1 1 1 1 1]
      | sbobj.Groups.Signals(11).Name = 'br'
      | sbobj.Groups.Signals(11).XData = [0 1 2 3 4 5 6 7 8 9 10 11 12 13 14 15 16 17 18 19 20]
      | sbobj.Groups.Signals(11).YData = [0 -1 -1 -1 -1 1 1 -1 -1 1 1 1 1 -1 1 1 1 1 1 1 1]
      | sbobj.Groups.Signals(12).Name = 'bl'
      | sbobj.Groups.Signals(12).XData = [0 1 2 3 4 5 6 7 8 9 10 11 12 13 14 15 16 17 18 19 20]
      | sbobj.Groups.Signals(12).YData = [0 -1 1 0 0 1 1 0 0 1 1 -1 -1 -1 -1 -1 -1 1 1 1 1]
      | sbobj.Groups.Signals(13).Name = 'l'
      | sbobj.Groups.Signals(13).XData = [0 1 2 3 4 5 6 7 8 9 10 11 12 13 14 15 16 17 18 19 20]
      | sbobj.Groups.Signals(13).YData = [0 0 0 0 0 0 1 1 1 1 1 1 1 0 0 0 0 0 0 0 0]
      | sbobj.Groups.Signals(14).Name = 'Internal Temp'
      | sbobj.Groups.Signals(14).XData = [0 1 2 3 4 5 6 7 8 9 10 11 12 13 14 15 16 17 18 19 20]
      | sbobj.Groups.Signals(14).YData = [5 10 15 20 25 30 30 5 10 15 20 25 30 30 5 10 15 20 25 30 30]
      | sbobj.Groups.Signals(15).Name = 'Engine Speed'
      | sbobj.Groups.Signals(15).XData = [0 1 2 3 4 5 6 7 8 9 10 11 12 13 14 15 16 17 18 19 20]
      | sbobj.Groups.Signals(15).YData = [0 20 40 60 80 100 120 0 20 40 60 80 100 120 0 20 40 60 80 100 120]
      | sbobj.Groups.Signals(16).Name = 'Comp Torque'
      | sbobj.Groups.Signals(16).XData = [0 1 2 3 4 5 6 7 8 9 10 11 12 13 14 15 16 17 18 19 20]
      | sbobj.Groups.Signals(16).YData = [5 10 15 20 25 30 30 5 10 15 20 25 30 30 5 10 15 20 25 30 30]
      | sbobj.Groups.Signals(17).Name = 'Blower Speed Proportional'
      | sbobj.Groups.Signals(17).XData = [0 1 2 3 4 5 6 7 8 9 10 11 12 13 14 15 16 17 18 19 20]
      | sbobj.Groups.Signals(17).YData = [2 2 4 6 8 10 12 2 2 4 6 8 10 12 2 2 4 6 8 10 12]
      | sbobj.Groups.TimeRange = [0 20]
  brake_input : Outport  Tag=STV Outport
  steering_angle : Outport  Tag=STV Outport  Port=2
  hazard_switch_input : Outport  Tag=STV Outport  Port=3
  key_input : Outport  Tag=STV Outport  Port=4
  gear_input : Outport  Tag=STV Outport  Port=5
  dw : Outport  Tag=STV Outport  Port=6
  fpd : Outport  Tag=STV Outport  Port=7
  brd : Outport  Tag=STV Outport  Port=8
  bld : Outport  Tag=STV Outport  Port=9
  fp : Outport  Tag=STV Outport  Port=10
  br : Outport  Tag=STV Outport  Port=11
  bl : Outport  Tag=STV Outport  Port=12
  l : Outport  Tag=STV Outport  Port=13
  Internal Temp : Outport  Tag=STV Outport  Port=14
  Engine Speed : Outport  Tag=STV Outport  Port=15
  Comp Torque : Outport  Tag=STV Outport  Port=16
  Blower Speed Proportional : Outport  Tag=STV Outport  Port=17
  wires:
  Demux/1 -> brake_input/1
  FromWs/1 -> Demux/1
  Demux/2 -> steering_angle/1
  Demux/3 -> hazard_switch_input/1
  Demux/4 -> key_input/1
  Demux/5 -> gear_input/1
  Demux/6 -> dw/1
  Demux/7 -> fpd/1
  Demux/8 -> brd/1
  Demux/9 -> bld/1
  Demux/10 -> fp/1
  Demux/11 -> br/1
  Demux/12 -> bl/1
  Demux/13 -> l/1
  Demux/14 -> Internal Temp/1
  Demux/15 -> Engine Speed/1
  Demux/16 -> Comp Torque/1
  Demux/17 -> Blower Speed Proportional/1

== system HilClimbers_Integrated_V8_2018b/variant_input_system/manual_inputs/INPUT ==
  blower_speed_proportion : Constant  Value=10
  engine_speed : Constant  Value=100
  engine_torque : Constant  Value=30
  internal_temperature : Constant  Value=28
  Internal_temperature : Outport
  Engine_speed : Outport  Port=2
  Engine_torque : Outport  Port=3
  Blower_speed_proportion : Outport  Port=4
  wires:
  internal_temperature/1 -> Internal_temperature/1
  engine_torque/1 -> Engine_torque/1
  blower_speed_proportion/1 -> Blower_speed_proportion/1
  engine_speed/1 -> Engine_speed/1

== system HilClimbers_Integrated_V8_2018b/variant_input_system/manual_inputs/manual_input_subsystem ==
  note: Inputs
  note: LRLM_inputs
  note: Inputs:
      | Brake Paddle
      | Steering
      | Hazard Light
      | Key
      | Gear
  Constant4 : Constant  Value=0
  Hazard_Light : SliderSwitchBlock  LabelPosition=Hide
      settings: Values={{'Off', 'On'}, [0 1]}
  Push Button : PushButtonBlock  ButtonText=Brake
  Radio Button : RadioButtonGroup  LabelPosition=Hide  SelectedLabel=Neutral  ButtonGroupName=Gear
      settings: Values={{'Neutral', 'Drive', 'Park', 'Reverse'}, [0 1 2 3]}
  Steering : KnobBlock  LabelPosition=Hide  ScaleMin=-90  ScaleMax=90  TickInterval=45
  brake_status : Constant  Value=0
  hazard_status : Constant  Value=0
  key_state : ToggleSwitchBlock  LabelPosition=Bottom
      settings: Values={{'Off', 'On'}, [0 1]}
  key_status : Constant
  steering : Constant  Value=0
  brake_input : Outport
  steering_angle : Outport  Port=2
  hazard_switch_input : Outport  Port=3
  key_input : Outport  Port=4
  gear_input : Outport  Port=5
  wires:
  brake_status/1 -> brake_input/1  "brake_input"
  Constant4/1 -> gear_input/1  "gear_input"
  steering/1 -> steering_angle/1  "steering_angle"
  key_status/1 -> key_input/1  "key_input"
  hazard_status/1 -> hazard_switch_input/1  "hazard_switch_input"

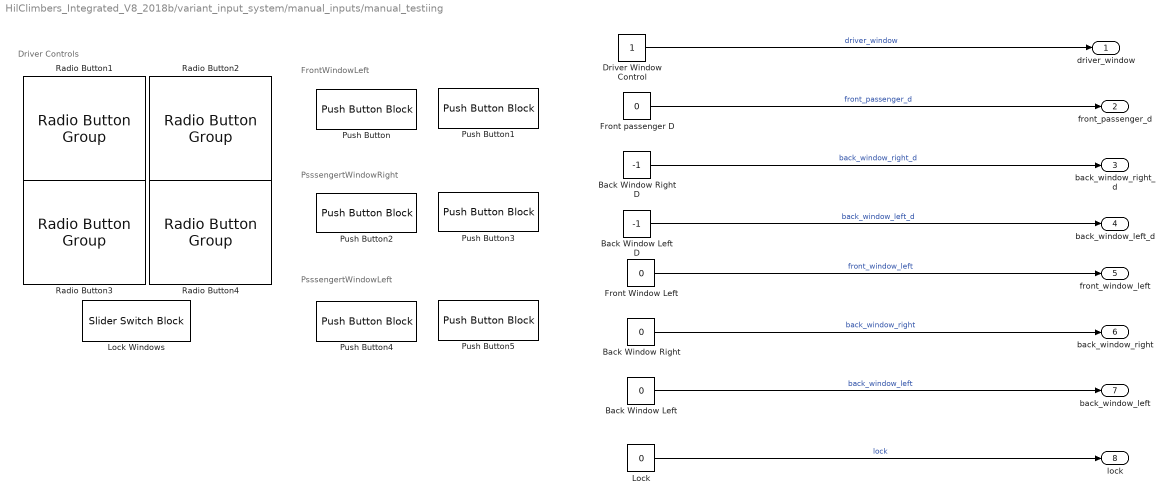
== system HilClimbers_Integrated_V8_2018b/variant_input_system/manual_inputs/manual_testiing ==
  note: PsssengertWindowLeft
  note: PsssengertWindowRight
  note: Driver Controls
  note: FrontWindowLeft
  Back Window Left : Constant  Value=0
  Back Window Left D : Constant  Value=-1
  Back Window Right : Constant  Value=0
  Back Window Right D : Constant  Value=-1
  Driver Window Control : Constant
  Front Window Left : Constant  Value=0
  Front passenger D : Constant  Value=0
  Lock : Constant  Value=0
  Lock Windows : SliderSwitchBlock
      settings: Values={{'Unlock', 'Lock'}, [0 1]}
  Push Button : PushButtonBlock  ButtonText=Push up window
  Push Button1 : PushButtonBlock  ButtonText=Pull down window  OnValue=-1
  Push Button2 : PushButtonBlock  ButtonText=Push up window
  Push Button3 : PushButtonBlock  ButtonText=Pull down window  OnValue=-1
  Push Button4 : PushButtonBlock  ButtonText=Push up window
  Push Button5 : PushButtonBlock  ButtonText=Pull down window  OnValue=-1
  Radio Button1 : RadioButtonGroup  LabelPosition=Hide  SelectedLabel=Open  ButtonGroupName=Driver Window Controls
      settings: Values={{'Open', 'Stop', 'Close'}, [1 0 -1]}
  Radio Button2 : RadioButtonGroup  LabelPosition=Hide  SelectedLabel=Stop  ButtonGroupName=Front Passenger
      settings: Values={{'Open', 'Stop', 'Close'}, [1 0 -1]}
  Radio Button3 : RadioButtonGroup  LabelPosition=Hide  SelectedLabel=Close  ButtonGroupName=Back Window Right
      settings: Values={{'Open', 'Stop', 'Close'}, [1 0 -1]}
  Radio Button4 : RadioButtonGroup  LabelPosition=Hide  SelectedLabel=Close  ButtonGroupName=Back Window Left
      settings: Values={{'Open', 'Stop', 'Close'}, [1 0 -1]}
  driver_window : Outport
  front_passenger_d : Outport  Port=2
  back_window_right_d : Outport  Port=3
  back_window_left_d : Outport  Port=4
  front_window_left : Outport  Port=5
  back_window_right : Outport  Port=6
  back_window_left : Outport  Port=7
  lock : Outport  Port=8
  wires:
  Front passenger D/1 -> front_passenger_d/1  "front_passenger_d"
  Lock/1 -> lock/1  "lock"
  Front Window Left/1 -> front_window_left/1  "front_window_left"
  Driver Window Control/1 -> driver_window/1  "driver_window"
  Back Window Right D/1 -> back_window_right_d/1  "back_window_right_d"
  Back Window Left/1 -> back_window_left/1  "back_window_left"
  Back Window Right/1 -> back_window_right/1  "back_window_right"
  Back Window Left D/1 -> back_window_left_d/1  "back_window_left_d"

== system HilClimbers_Integrated_V8_2018b/main_ECU/LRLM_ECU/indicator_system/left_indicator_system ==
  steering_angle : Inport
  hazard_status : Inport  Port=2
  If2 : If  NumInputs=2  IfExpression=u1 < 0 | u2 ==1
  indictator_light_output_decider : BCM/indictator_light_output_decider
      settings: SourceProductName=BCM Library
  left_indicator_signal : Outport
  wires:
  hazard_status/1 -> If2/2  "hazard_status"
  steering_angle/1 -> If2/1  "steering_angle"
  If2/1 -> indictator_light_output_decider/1
  indictator_light_output_decider/1 -> left_indicator_signal/1  "left_indicator_signal"
  If2/2 -> indictator_light_output_decider/2

== system HilClimbers_Integrated_V8_2018b/main_ECU/LRLM_ECU/indicator_system/right_indicator_system ==
  steering_angle : Inport
  hazard_status : Inport  Port=2
  If1 : If  NumInputs=2  IfExpression=u1 > 0 | u2 ==1
  indictator_light_output_decider : BCM/indictator_light_output_decider
      settings: SourceProductName=BCM Library
  right_indicator_signal : Outport
  wires:
  hazard_status/1 -> If1/2  "hazard_status"
  steering_angle/1 -> If1/1  "steering_angle"
  If1/1 -> indictator_light_output_decider/1
  indictator_light_output_decider/1 -> right_indicator_signal/1  "right_indicator_signal"
  If1/2 -> indictator_light_output_decider/2

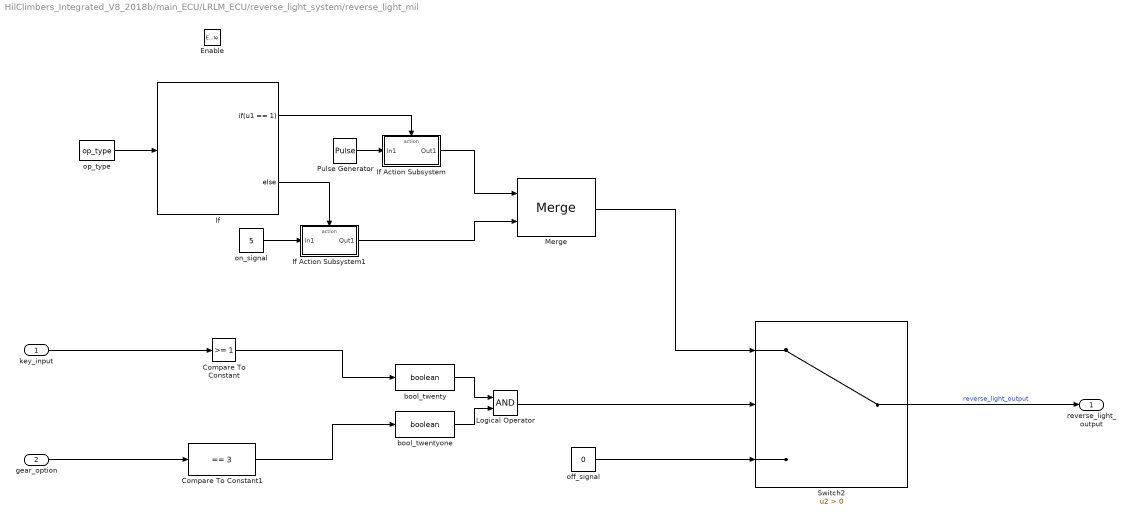
== system HilClimbers_Integrated_V8_2018b/main_ECU/LRLM_ECU/reverse_light_system/reverse_light_mil ==
  key_input : Inport
  gear_option : Inport  Port=2
  Enable : EnablePort  StatesWhenEnabling=reset
  Compare To Constant : simulink/Logic and Bit Operations/Compare To Constant  relop=>=  const=1  OutDataTypeStr=boolean
  Compare To Constant1 : simulink/Logic and Bit Operations/Compare To Constant  relop===  const=3  OutDataTypeStr=boolean
  If : If  IfExpression=u1 == 1
  If Action Subsystem : Subsystem  TreatAsAtomicUnit=on
  If Action Subsystem1 : Subsystem  TreatAsAtomicUnit=on
  Logical Operator : Logic  AllPortsSameDT=off  OutDataTypeStr=boolean
  Merge : Merge
  Pulse Generator : DiscretePulseGenerator  PulseType=Time based  Amplitude=5  Period=0.1  PulseWidth=5
  Switch2 : Switch  Criteria=u2 > Threshold
  bool_twenty : DataTypeConversion  OutDataTypeStr=boolean
  bool_twentyone : DataTypeConversion  OutDataTypeStr=boolean
  off_signal : Constant  Value=0
  on_signal : Constant  Value=5
  op_type : Constant  Value=op_type
  reverse_light_output : Outport
  wires:
  Compare To Constant1/1 -> bool_twentyone/1
  Switch2/1 -> reverse_light_output/1  "reverse_light_output"
  op_type/1 -> If/1
  If/2 -> If Action Subsystem1/Action
  If Action Subsystem/1(Out1) -> Merge/1
  bool_twentyone/1 -> Logical Operator/2
  on_signal/1 -> If Action Subsystem1/1(In1)
  Pulse Generator/1 -> If Action Subsystem/1(In1)
  If/1 -> If Action Subsystem/Action
  key_input/1 -> Compare To Constant/1
  Compare To Constant/1 -> bool_twenty/1
  If Action Subsystem1/1(Out1) -> Merge/2
  Merge/1 -> Switch2/1
  off_signal/1 -> Switch2/3
  bool_twenty/1 -> Logical Operator/1
  gear_option/1 -> Compare To Constant1/1
  Logical Operator/1 -> Switch2/2

== system HilClimbers_Integrated_V8_2018b/main_ECU/LRLM_ECU/reverse_light_system/reverse_light_sil ==
  key_input : Inport
  gear_option : Inport  Port=2
  Enable : Inport  Port=3
  Enabled Subsystem_sfcn : S-Function  FunctionName=Enabled_sf  Parameters=sfcnParam1  SFunctionModules=""  SFunctionDeploymentMode=off  EnableBusSupport=off  mask{rtw_sf_name=Enabled_sf, showVar=off, sfcnParam1=sfcnParam1}
      mask prompts: rtw_sf_name "Simulink:masks:GenSFuncName_MP"; showVar "Simulink:masks:GenSFuncShowModuleList_MP"; sfcnParam1 "op_type:"
      mask help: Simulink:masks:GenSFuncDesc_MD
      mask init:
      | displist = '';
      | if ~strcmp(get_param(gcb, 'FunctionName'), rtw_sf_name);
      |   set_param(gcb, 'FunctionName', rtw_sf_name);
      | end
      | % Check if we are generating code
      | rtw_mode = false;
      | if strcmpi(get_param(bdroot(gcb),'SimulationStatus'),'Initializing')
      | 	rtw_mode = strcmpi(get_param(bdroot(gcb),'BuildingRTWCode'),'on') && ...
      | 		~strcmpi(get_param(bdroot(gcb),'TargetStyle'),'SimulationTarget');
      | end
      | if showVar || rtw_mode
      | 	if exist('rtwsfunc') == 2 | exist('rtwsfunc') == 6
      | 		tmplist = rtwsfunc(rtw_sf_name,gcb);
      | 		tmplist = DAStudio.message('Simulink:masks:GenSFuncListOfModules_IC', tmplist);
      | 	elseif showVar
      | 		tmplist1 = DAStudio.message('Simulink:masks:GenSFuncListOfModules_IC', '');
      |         tmplist2 = DAStudio.message('Simulink:masks:GenSFuncNotLicensed_IC');
      |         tmplist = [tmplist1 tmplist2];
      |  	end
      | end
      | if showVar
      |   displist = tmplist;
      | end
      settings: CopyFcn=|
      | if ~strcmp(get_param(gcb,'Linkstatus'),'none') && ...
      | ~strcmp(get_param(gcb,'Linkstatus'),'implicit')
      |   set_param(gcb,'LinkStatus','none');
      | end
      mask Help: eval('feval(''rtwprivate'',''rtwhelpview'',''rtw_sfcn_block'')');
      mask Display:
      | port_label('input',1,'key_input');
      | port_label('input',2,'gear_option');
      | port_label('input',3,'Enable');
      | port_label('output',1,'reverse_light_output');
  __InputSSForSFun__ : Subsystem
  __OutputSSForSFun__ : Subsystem
  reverse_light_output : Outport
  wires:
  key_input/1 -> __InputSSForSFun__/1(key_input)
  gear_option/1 -> __InputSSForSFun__/2(gear_option)
  Enable/1 -> __InputSSForSFun__/3(Enable)
  __InputSSForSFun__/1(__UniqueOutportName__1__) -> Enabled Subsystem_sfcn/1
  __InputSSForSFun__/2(__UniqueOutportName__2__) -> Enabled Subsystem_sfcn/2
  __InputSSForSFun__/3(__UniqueOutportName__3__) -> Enabled Subsystem_sfcn/3
  Enabled Subsystem_sfcn/1 -> __OutputSSForSFun__/1(__UniqueInportName__1__)
  __OutputSSForSFun__/1(reverse_light_output) -> reverse_light_output/1

== system HilClimbers_Integrated_V8_2018b/main_ECU/LRLM_ECU/reverse_light_system/reverse_light_mil/If Action Subsystem ==
  In1 : Inport
  Action Port : ActionPort
  Out1 : Outport
  wires:
  In1/1 -> Out1/1

== system HilClimbers_Integrated_V8_2018b/main_ECU/LRLM_ECU/reverse_light_system/reverse_light_mil/If Action Subsystem1 ==
  In1 : Inport
  Action Port : ActionPort
  Out1 : Outport
  wires:
  In1/1 -> Out1/1

== system HilClimbers_Integrated_V8_2018b/main_ECU/LRLM_ECU/reverse_light_system/reverse_light_sil/__InputSSForSFun__ ==
  key_input : Inport
  gear_option : Inport  Port=2
  Enable : Inport  Port=3
  __UniqueOutportName__1__ : Outport
  __UniqueOutportName__2__ : Outport  Port=2
  __UniqueOutportName__3__ : Outport  Port=3
  wires:
  key_input/1 -> __UniqueOutportName__1__/1
  gear_option/1 -> __UniqueOutportName__2__/1
  Enable/1 -> __UniqueOutportName__3__/1

== system HilClimbers_Integrated_V8_2018b/main_ECU/LRLM_ECU/reverse_light_system/reverse_light_sil/__OutputSSForSFun__ ==
  __UniqueInportName__1__ : Inport
  reverse_light_output : Outport
  wires:
  __UniqueInportName__1__/1 -> reverse_light_output/1  "reverse_light_output"

== matlab function HilClimbers_Integrated_V8_2018b/main_ECU/power_window_ECU/MATLAB Function4 ==
  data: dw input double size=1; Va_d output double size=1; front_passenger input double size=1; back_passenger_right input double size=1; back_passenger_left input double size=1; Va_fpd output double size=1; Va_bpr output double size=1; Va_bpl output double size=1
function [Va_d,Va_fpd, Va_bpr, Va_bpl] = fcn(dw, front_passenger, back_passenger_right, back_passenger_left)
dout=0;
fpd=0;
bpr=0;
bpl=0;
if (dw==1)
    dout=20;
elseif (dw==-1)
    dout=-20;
elseif (dw==0)
    dout=0;
end

if (front_passenger==1)
        fpd=20;
elseif (front_passenger==-1)
    fpd=-20;
elseif (front_passenger==0)
    fpd=0;
end

if (back_passenger_right==1)
        bpr=20;
elseif (back_passenger_right==-1)
    bpr=-20;
elseif (back_passenger_right==0)
    bpr=0;
end

if (back_passenger_left==1)
        bpl=20;
elseif (back_passenger_left==-1)
    bpl=-20;
elseif (back_passenger_left==0)
    bpl=0;
end
  
Va_d = dout;
Va_fpd = fpd;
Va_bpr=bpr;
Va_bpl=bpl;

== matlab function HilClimbers_Integrated_V8_2018b/systems_and_impact/Subsystem Reference/MATLAB Function ==
  data: pr input double size=1; pr_o output double size=1; d_o output double size=1; d input double size=1; pl input double size=1; fp input double size=1; pl_o output double size=1; fp_o output double size=1
function [pr_o,d_o,pl_o, fp_o] = fcn(pr, d, pl, fp)
if pr>=10
    prout=10;
elseif pr<=0
    prout=0;
else
    prout=pr;
end

if d>=10
    dout=10;
elseif d<=0
    dout=0;
else
    dout=d;
end

if pl>=10
    plout=10;
elseif pl<=0
    plout=0;
else
    plout=pr;
end

if fp>=10
    fpout=10;
elseif fp<=0
    fpout=0;
else
    fpout=fp;
end
pr_o=prout;
d_o=dout;
pl_o=plout;
fp_o=fpout;
